simulink model "Diode_Model"  (R2020b)
settings: Solver=FixedStepDiscrete  StartTime=0.0  StopTime=10.0  RelTol=1e-3
libraries: powerlib x7
settings Model: Creator=vijay jagtap  LastModifiedBy=vijay jagtap

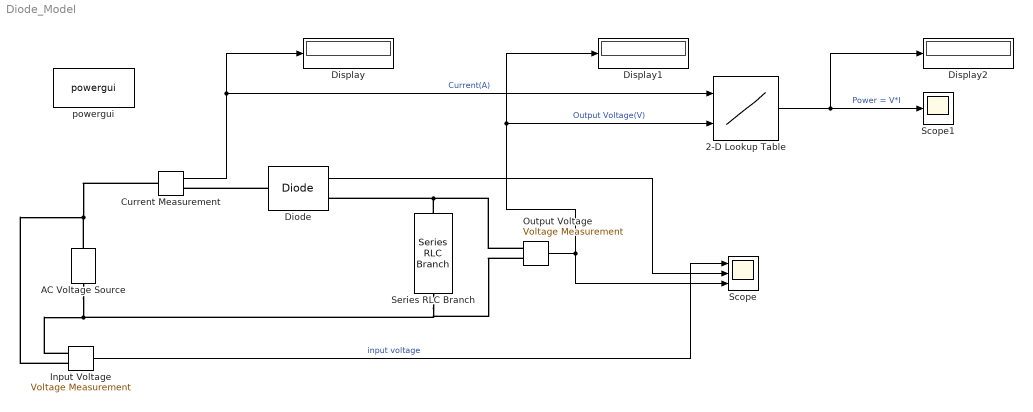
== system Diode_Model ==
  2-D Lookup Table : Lookup_n-D  BreakpointsForDimension1=[1,2,3]  BreakpointsForDimension2=[1,2,3]  Table=reshape([1,2,3,2,4,6,3,6,9],3,3)  InternalRulePriority=Speed  RndMeth=Simplest  InputSameDT=on
      settings: InputPortMap=u0,u1
  AC Voltage Source : powerlib/Electrical Sources/AC Voltage Source  Amplitude=220  Phase=0  Frequency=60  SampleTime=-1  Measurements=None  BusType=swing  Pref=10e3  Qref=0  Qmin=-inf  Qmax=+inf
  Current Measurement : powerlib/Measurements/Current Measurement  PhasorSimulation=off  OutputType=Complex  PSBequivalent=0
  Diode : powerlib/Power Electronics/Diode  Ron=0.001  Lon=0  Vf=0.8  IC=0  UseSnubber=0  Rs=500  Cs=250e-9  Measurements=on
  Display : Display
  Display1 : Display
  Display2 : Display
  Input Voltage : powerlib/Measurements/Voltage Measurement  PhasorSimulation=off  OutputType=Complex  PSBequivalent=0
  Output Voltage : powerlib/Measurements/Voltage Measurement  PhasorSimulation=off  OutputType=Complex  PSBequivalent=0
  Scope : Scope  NumInputPorts=3
  Scope1 : Scope
  Series RLC Branch : powerlib/Elements/Series RLC Branch  LConnTagsString=__new0  RConnTagsString=__new0  BranchType=R  Resistance=1000  Inductance=1e-3  SetiL0=off  InitialCurrent=0  Capacitance=1e-6  Setx0=off  InitialVoltage=0  Measurements=None
  powergui : powerlib/powergui  Priority=1  SimulationMode=Discrete  SampleTime=50e-6  frequency=60  Iterations=50  frequencyindice=60  Pbase=100e6  ErrMax=1e-4  UnitsV=kV  UnitsW=MW  buscounter=0  FunctionMessages=off  echomessages=off  EnableUseOfTLC=off  CurrentSourceSwitches=off  DisableSnubberDevices=off  DisableRonSwitches=off  DisableVfSwitches=off  DisplayEquations=off  AutomaticDiscreteSolvers=off  SolverType=Tustin/Backward Euler (TBE)  Interpol=off  ExternalGateDelay=off  methode=off  Ts=100  x0status=blocks  SPID=on  SwTol=0  HookPort=off  NonlinearTolerance=1e-4  nMaxIteration=100  ContinueOnMaxIteration=off  RestoreLinks=warning  ResistiveCurrentMeasurement=off  Frange=[0:2:500]  Ylog=off  Xlog=on  ShowGrid=off  save=off  variable=ZData  structure=0  ZoomFFT=off  StartTime=0.0  cycles=1  DisplayStyle=1  fundamental=60  FreqAxis=off  MaxFrequency=1000  frequencyindicesteady=1  RmsSteady=1  display=off
  wires:
  Output Voltage/1 -> Display1/1, 2-D Lookup Table/2, Scope/3  "Output Voltage(V)"
  Current Measurement/1 -> 2-D Lookup Table/1, Display/1  "Current(A)"
  Diode/1 -> Scope/2
  2-D Lookup Table/1 -> Display2/1, Scope1/1  "Power = V*I"
  Input Voltage/1 -> Scope/1  "input voltage"
  connections:
  Output Voltage/LConn1 -- Series RLC Branch/LConn1 -- Diode/RConn1
  Input Voltage/LConn2 -- Series RLC Branch/RConn1 -- Output Voltage/LConn2 -- AC Voltage Source/LConn1
  Input Voltage/LConn1 -- Current Measurement/LConn1 -- AC Voltage Source/RConn1
  Diode/LConn1 -- Current Measurement/RConn1
